simulink model "LKAS_AutoSave_20220223_1234"  (R2018b)
settings: Solver=FixedStepDiscrete  StartTime=0.0  StopTime=10.0  FixedStep=0.01  RelTol=1e-3
InitFcn:
  | tmpVer = ver('MATLAB');
  | tmpVer = str2num(tmpVer.Version);
  | % -------------------------------------------------------------------
  | %  MATLAB file generated by Simulink.saveVars on 21-Nov-2019 10:06:14
  | %  MATLAB version: 7.13.0.564 (R2011b)
  | % -------------------------------------------------------------------
  | 
  | 
  | SInt16 = Simulink.AliasType;
  | SInt16.Description = 'Num';
  | if (tmpVer > 7.11)
  | 	SInt16.DataScope = 'Auto';
  | end
  | SInt16.HeaderFile = 'Rte_Type.h';
  | SInt16.BaseType = 'int16';
  | 
  | SInt32 = Simulink.AliasType;
  | SInt32.Description = 'Num';
  | if (tmpVer > 7.11)
  | 	SInt32.DataScope = 'Auto';
  | end
  | SInt32.HeaderFile = 'Rte_Type.h';
  | SInt32.BaseType = 'int32';
  | 
  | SInt8 = Simulink.AliasType;
  | SInt8.Description = 'Num';
  | if (tmpVer > 7.11)
  | 	SInt8.DataScope = 'Auto';
  | end
  | SInt8.HeaderFile = 'Rte_Type.h';
  | SInt8.BaseType = 'int8';
  | 
  | T_A_m2_1024_1_u32 = Simulink.NumericType;
  | T_A_m2_1024_1_u32.Description = 'm2 (square meters  (m2))';
  | if (tmpVer > 7.11)
  | 	T_A_m2_1024_1_u32.DataScope = 'Auto';
  | end
  | T_A_m2_1024_1_u32.HeaderFile = 'Rte_Type.h';
  | T_A_m2_1024_1_u32.DataTypeMode = 'Fixed-point: slope and bias scaling';
  | T_A_m2_1024_1_u32.SignednessBool = false;
  | T_A_m2_1024_1_u32.WordLength = 32;
  | T_A_m2_1024_1_u32.FixedExponent = -10;
  | T_A_m2_1024_1_u32.SlopeAdjustmentFactor = 1;
  | T_A_m2_1024_1_u32.Bias = 0;
  | T_A_m2_1024_1_u32.DataTypeOverride = 'Inherit';
  | T_A_m2_1024_1_u32.IsAlias = true;
  | 
  | T_A_m2_65536_1_u16 = Simulink.NumericType;
  | T_A_m2_65536_1_u16.Description = 'm2 (square meters  (m2))';
  | if (tmpVer > 7.11)
  | 	T_A_m2_65536_1_u16.DataScope = 'Auto';
  | end
  | T_A_m2_65536_1_u16.HeaderFile = 'Rte_Type.h';
  | T_A_m2_65536_1_u16.DataTypeMode = 'Fixed-point: slope and bias scaling';
  | T_A_m2_65536_1_u16.SignednessBool = false;
  | T_A_m2_65536_1_u16.WordLength = 16;
  | T_A_m2_65536_1_u16.FixedExponent = -16;
  | T_A_m2_65536_1_u16.SlopeAdjustmentFactor = 1;
  | T_A_m2_65536_1_u16.Bias = 0;
  | T_A_m2_65536_1_u16.DataTypeOverride = 'Inherit';
  | ... (+4647 lines)
StopFcn:
  | clear  T_A_m2_1024_1_u32 T_A_m2_65536_1_u16 T_A_m2_Float32 T_A_mm2_10_1_u16 T_A_mm2_4_1_s16 T_A_mm2_Float32 T_Cnt_Num_10_1_u32 T_Cnt_Num_1_1_s16 T_Cnt_Num_1_1_s32 T_Cnt_Num_1_1_s8 T_Cnt_Num_1_1_u16 T_Cnt_Num_1_1_u32 T_Cnt_Num_1_1_u8 T_E_J_1_1_s32 T_E_J_Float32 T_E_kJ_128_1_s32 T_E_kJ_Float32 T_E_kwh_10_1_u16 T_E_kwh_Float32 T_Epl_kwhpkm_100_1_u16 T_Epl_kwhpkm_Float32 T_F_N_1_1_s16 T_F_N_Float32 T_I_A_1000_1_u16 T_I_A_1048576_1_s32 T_I_A_2048_1_s16 T_I_A_32_1_s16 T_I_A_Float32 T_I_mA_1_1_s16 T_I_mA_32768_128_s16 T_I_mA_Float32 T_J_kgpm2_128_1_u16 T_J_kgpm2_Float32 T_K_NA_1000_1_s16 T_K_NA_100_1_s16 T_K_NA_100_1_u16 T_K_NA_1024_1_s16 T_K_NA_1024_1_u16 T_K_NA_128_1_s16 T_K_NA_128_1_u16 T_K_NA_128_1_u8 T_K_NA_16777216_1_u32 T_K_NA_16_1_s16 T_K_NA_16_1_u16 T_K_NA_16_1_u8 T_K_NA_1_16_u16 T_K_NA_1_1_s16 T_K_NA_1_1_u16 T_K_NA_1_1_u8 T_K_NA_32768_1_s16 T_K_NA_32768_1_u16 T_K_NA_32_1_s8 T_K_NA_4096_1_u16 T_K_NA_4194304_1_s32 T_K_NA_4194304_1_u16 T_K_NA_65536_1_s32 T_K_NA_65536_1_u16 T_K_NA_8192_1_s16 T_K_NA_8_1_s16 T_K_NA_Float32 T_M_Nm_16_1_s16 T_M_Nm_1_1_s16 T_M_Nm_32768_1_s16 T_M_Nm_32_1_s16 T_M_Nm_4_1_s16 T_M_Nm_512_1_s16 T_M_Nm_Float32 T_P_W_1_4_s16 T_P_W_1_8_s16 T_P_W_Float32 T_P_kW_128_1_s16 T_P_kW_1_8_s16 T_P_kW_8_1_s32 T_P_kW_Float32 T_Pct_pct_1024_1_s32 T_Pct_pct_1024_1_u32 T_Pct_pct_10_1_s16 T_Pct_pct_10_1_u32 T_Pct_pct_128_100_s8 T_Pct_pct_1_1_s16 T_Pct_pct_1_4_u8 T_Pct_pct_255_100_u16 T_Pct_pct_255_100_u8 T_Pct_pct_256_1_s16 T_Pct_pct_256_1_u16 T_Pct_pct_65535_100_u16 T_Pct_pct_Float32 T_R_ohm_1024_1_s16 T_R_ohm_32_1_s16 T_R_ohm_Float32 T_TK_K_16_1_s16 T_TK_K_Float32 T_T_degC_10_400_1_u16 T_T_degC_16_1_s16 T_T_degC_1_40_1_u8 T_T_degC_2_80_1_u8 T_T_degC_Float32 T_U_V_1000_1_u16 T_U_V_10_1_u8 T_U_V_200_1_u8 T_U_V_32_1_s16 T_U_V_4096_1_s16 T_U_V_512_1_s16 T_U_V_65535_8_u16 T_U_V_8192_1_u16 T_U_V_Float32 T_U_mV_1_1_s16 T_U_mV_256_20_u16 T_U_mV_Float32 T_V_l_256_1_s16 T_V_l_4096_1_s16 T_V_l_64_1_s16 T_V_l_65535_100_u16 T_V_l_Float32 T_V_ml_128_1_s16 T_V_ml_1_1_s16 T_V_ml_32768_1_s16 T_V_ml_Float32 T_V_ul_32_1_u16 T_V_ul_Float32 T_Vpl_clpkm_512_1_u16 T_Vpl_clpkm_Float32 T_a_kphps_16_1_s16 T_a_kphps_Float32 T_a_mps2_128_1_s16 T_a_mps2_Float32 T_c_MJpkg_256_1_s16 T_c_MJpkg_Float32 T_c_kJpgpK_1024_1_s16 T_c_kJpgpK_Float32 T_c_kJpkgpK_128_1_u16 T_c_kJpkgpK_Float32 T_chrg_Ah_1_1_s16 T_chrg_Ah_1_1_u16 T_chrg_Ah_1_1_u8 T_chrg_Ah_256_1_u16 T_chrg_Ah_4194304_1_s32 T_chrg_Ah_512_1_u16 T_chrg_Ah_8_1_u16 T_chrg_Ah_Float32 T_cmp_NA_100_1_s16 T_cmp_NA_128_1_s16 T_cmp_NA_16_1_s16 T_cmp_NA_32768_1_u16 T_cmp_NA_Float32 T_d2n_rpmps2_4_1_s16 T_d2n_rpmps2_Float32 T_dPct_pctps_16_1_s16 T_dPct_pctps_256_1_s16 T_dPct_pctps_Float32 T_dT_degCps_128_1_s16 T_dT_degCps_Float32 T_dV_lph_1_1_s16 T_dV_lph_Float32 T_dV_lpm_128_1_s16 T_dV_lpm_32_1_s16 T_dV_lpm_Float32 T_dV_lps_1024_1_u16 T_dV_lps_4_1_u16 T_dV_lps_Float32 T_dV_mlps_1024_1_s16 T_dV_mlps_Float32 T_d_BitField16 T_dm_gps_128_1_s16 T_dm_gps_128_1_u16 T_dm_gps_256_1_u16 T_dm_gps_Float32 T_dm_mgps_1_1_s16 T_dm_mgps_Float32 T_dn_rpmps_1_1_s16 T_dn_rpmps_2_1_s16 T_dn_rpmps_Float32 T_dp_Paps_1_1_s16 T_dp_Paps_Float32 T_dp_kPaps_1_1_s16 T_dp_kPaps_8_1_s16 T_dp_kPaps_Float32 T_dphi_degps_128_1_s16 T_dphi_degps_8_1_s16 T_dphi_degps_Float32 T_dr_ps_256_1_s16 T_dr_ps_Float32 T_drho_mgplps_1_2_s16 T_drho_mgplps_Float32 T_e_NA_1_1_u8 T_f_Hz_1_1_u16 T_f_Hz_1_1_u32 T_f_Hz_64_1_u16 T_f_Hz_8_1_s16 T_f_Hz_Float32 T_g_BitField32 T_l_km_16_1_s16 T_l_km_1_1_u16 T_l_km_1_1_u32 T_l_km_Float32 T_l_m_1024_1_s16 T_l_m_16_1_s16 T_l_m_1_1_u32 T_l_m_Float32 T_l_mm_16_1_s16 T_l_mm_1_1_u16 T_l_mm_4096_1_s16 T_l_mm_4_1_u8 T_l_mm_64_1_s16 T_l_mm_Float32 T_m_g_1_1_s16 T_m_g_2048_1_s16 T_m_g_32_1_u16 T_m_g_Float32 T_m_kg_1024_1_s16 T_m_kg_1_1_s16 T_m_kg_1_1_u32 T_m_kg_Float32 T_m_mg_128_1_s16 T_m_mg_32_1_s16 T_m_mg_Float32 T_n_rpm_1_1_s16 T_n_rpm_1_25_u8 T_n_rpm_256_50_u16 T_n_rpm_2_25_u8 T_n_rpm_4_1_u16 T_n_rpm_Float32 T_p_MPa_64_1_s16 T_p_MPa_Float32 T_p_Pa_1_1_s16 T_p_Pa_Float32 T_p_kPa_1_10_u16 T_p_kPa_1_1_s16 T_p_kPa_1_1_u8 T_p_kPa_256_1_u16 T_p_kPa_32_1_u16 T_p_kPa_64_1_s16 T_p_kPa_Float32 T_phi_deg_100_1_s16 T_phi_deg_1024_1_s16 T_phi_deg_128_1_s16 T_phi_deg_1_1_u8 T_phi_deg_256_1_s16 T_phi_deg_2_1_s8 T_phi_deg_32_1_s16 T_phi_deg_512_6_s32 T_phi_deg_Float32 T_phi_rad_2048_1_s16 T_phi_rad_Float32 T_r_NA_1024_1_s16 T_r_NA_1024_1_u16 T_r_NA_16384_1_s16 T_r_NA_16_1_s16 T_r_NA_256_1_s8 T_r_NA_256_1_u16 T_r_NA_32768_1_u16 T_r_NA_32_1_u16 T_r_NA_4096_1_s16 T_r_NA_65535_2_u16 T_r_NA_8192_1_u16 T_r_NA_Float32 T_rho_gpl_8192_1_s16 T_rho_gpl_Float32 T_rho_kgpm3_16_1_s16 T_rho_kgpm3_Float32 T_rho_mgpl_1_1_s16 T_rho_mgpl_64_1_s16 T_rho_mgpl_Float32 T_t_hour_1_1_s16 T_t_hour_Float32 T_t_m_1_1_u16 T_t_m_Float32 T_t_ms_1_1_s16 T_t_ms_1_1_u16 T_t_ms_1_1_u32 T_t_ms_4096_1_s16 T_t_ms_64_1_s16 T_t_ms_Float32 T_t_s_1000_1_s16 T_t_s_100_1_s16 T_t_s_10_1_s16 T_t_s_10_1_u16 T_t_s_1_1_s16 T_t_s_1_1_u16 T_t_s_1_1_u32 T_t_s_Float32 T_t_us_10_1_u32 T_t_us_1_1_s16 T_t_us_1_1_u32 T_t_us_1_4_u16 T_t_us_Float32 T_v_kph_1_1_u8 T_v_kph_64_1_s16 T_v_kph_64_1_u16 T_v_kph_Float32 T_v_mps_256_1_s16 T_v_mps_Float32 T_w_radps_32_1_s16 T_w_radps_Float32 T_y_BitField8 T_y_BitFieldDiagProgress T_y_BitFieldDiagStatus T_y_NA_1_1_u8 SInt16 SInt32 SInt8 T_BOOLEAN UInt16 UInt32 UInt8 s16 s32 s8 u16 u32 u8
model workspace (MAT data in the model file):
  MCOS : class17 (value not decoded)
  MCOS : class17 (value not decoded)
  MCOS : class17 (value not decoded)
  MCOS : class17 (value not decoded)
  MCOS : class17 (value not decoded)
  MCOS : class17 (value not decoded)
  MCOS : class17 (value not decoded)
  MCOS : class17 (value not decoded)
  MCOS : class17 (value not decoded)
  MCOS : class17 (value not decoded)
  MCOS : class17 (value not decoded)
  MCOS : class17 (value not decoded)
  MCOS : class17 (value not decoded)
  MCOS : class17 (value not decoded)
  MCOS : class17 (value not decoded)
  MCOS : class17 (value not decoded)
  MCOS : class17 (value not decoded)
  MCOS : class17 (value not decoded)
  MCOS : class17 (value not decoded)
  MCOS : class17 (value not decoded)
  MCOS : class17 (value not decoded)
  MCOS : class17 (value not decoded)
  MCOS : class17 (value not decoded)
  MCOS : class17 (value not decoded)
  MCOS : class17 (value not decoded)
  MCOS : class17 (value not decoded)
  MCOS : class17 (value not decoded)
  MCOS : class17 (value not decoded)
  MCOS : class17 (value not decoded)
  MCOS : class17 (value not decoded)
  MCOS : class17 (value not decoded)
  MCOS : class17 (value not decoded)
  MCOS : class17 (value not decoded)
  MCOS : class17 (value not decoded)
  MCOS : class17 (value not decoded)
  MCOS : class17 (value not decoded)
  MCOS : class17 (value not decoded)
  MCOS : class17 (value not decoded)
  MCOS : class17 (value not decoded)
  MCOS : class17 (value not decoded)
  MCOS : class17 (value not decoded)
  MCOS : class17 (value not decoded)
  MCOS : class17 (value not decoded)
  MCOS : class17 (value not decoded)
  MCOS : class17 (value not decoded)
  MCOS : class17 (value not decoded)
  MCOS : class17 (value not decoded)
  MCOS : class17 (value not decoded)
  MCOS : class17 (value not decoded)
  MCOS : class17 (value not decoded)
  MCOS : class17 (value not decoded)
  MCOS : class17 (value not decoded)
  MCOS : class17 (value not decoded)
  MCOS : class17 (value not decoded)
  MCOS : class17 (value not decoded)
  MCOS : class17 (value not decoded)
  MCOS : class17 (value not decoded)
  MCOS : class17 (value not decoded)
  MCOS : class17 (value not decoded)
  MCOS : class17 (value not decoded)
  MCOS : class17 (value not decoded)
  MCOS : class17 (value not decoded)
  MCOS : class17 (value not decoded)
  MCOS : class17 (value not decoded)
  MCOS : class17 (value not decoded)
  MCOS : class17 (value not decoded)
  MCOS : class17 (value not decoded)
  MCOS : class17 (value not decoded)
  MCOS : class17 (value not decoded)
  MCOS : class17 (value not decoded)
  MCOS : class17 (value not decoded)
  MCOS : class17 (value not decoded)
  MCOS : class17 (value not decoded)
  MCOS : class17 (value not decoded)
  MCOS : class17 (value not decoded)
  MCOS : class17 (value not decoded)
  MCOS : class17 (value not decoded)
  MCOS : class17 (value not decoded)
  MCOS : class17 (value not decoded)
  MCOS : class17 (value not decoded)
  MCOS : class17 (value not decoded)
  MCOS : class17 (value not decoded)
  MCOS : class17 (value not decoded)
  MCOS : class17 (value not decoded)
  MCOS : class17 (value not decoded)
  MCOS : class17 (value not decoded)
  MCOS : class17 (value not decoded)
  MCOS : class17 (value not decoded)
  MCOS : class17 (value not decoded)
  MCOS : class17 (value not decoded)
  MCOS : class17 (value not decoded)
  MCOS : class17 (value not decoded)
  MCOS : class17 (value not decoded)
  MCOS : class17 (value not decoded)
  MCOS : class17 (value not decoded)
  MCOS : class17 (value not decoded)
  MCOS : class17 (value not decoded)
  MCOS : class17 (value not decoded)
  MCOS : class17 (value not decoded)
  MCOS : class17 (value not decoded)
  MCOS : class17 (value not decoded)
  MCOS : class17 (value not decoded)
undefined symbols (not defined in the file): LKA_CarWidth, LKA_SampleTime, LKA_StrRatio_C, LKA_Veh2CamL_C, LKA_Veh2CamW_C, LKA_WhlBaseL_C, LL_CompHdAg_C, LL_CompSWA_C, LL_CrvtPrvwT_C, LL_DesDvt_C, LL_DvtComp_C, LL_DvtPrvwT_C, LL_DvtSpdDet_vDvtSpdMin_C, LL_HandsOff_ExitTime, LL_HandsOff_TextTime, LL_HandsOff_WarnTime, LL_HdAgExT_C, LL_HdAgPrvwT_C, LL_LAccMax_C, LL_LAccRMax_C, LL_LDW_EarliestWarnLine_C, LL_LDW_LatestWarnLine_C, LL_LDWS_SUPPRESS_HEADING, LL_LFClb_TFC_FfCtlRatio_C, LL_LFClb_TFC_KdBalance_C, LL_LFClb_TFC_KdMaxSWA_C, LL_LFClb_TFC_KdV1_C, LL_LFClb_TFC_KdV2_C, LL_LFClb_TFC_KdVehSpdLwr_C, LL_LFClb_TFC_KdVehSpdUpr_C, LL_LFClb_TFC_Ki_C, LL_LFClb_TFC_KiMaxSWA_C, LL_LFClb_TFC_Kp_C, LL_LFClb_TFC_KpKlat_C, LL_LFClb_TFC_KpV1_C, LL_LFClb_TFC_KpV2_C, LL_LFClb_TFC_KpVehSpdLwr_C, LL_LFClb_TFC_KpVehSpdUpr_C, LL_LFClb_TFC_PrvwT_C, LL_LKA_EarliestWarnLine_C, LL_LKA_LatestWarnLine_C, LL_LKAExPrcs_ExitC0Dvt, LL_LKAExPrcs_ExitC0Swt, LL_LKAExPrcs_tiExitTime1, LL_LKAExPrcs_tiExitTime2, LL_LKAExPrcs_tiExitTime3, LL_LKAS_OUT_OF_CONTROL_LAT_VEL, LL_LKAS_OUT_OF_CONTROL_TTLC, LL_LKASWASyn_M0, LL_LKASWASyn_M1, LL_LKASWASyn_M2, LL_LKASWASyn_M3K, LL_LKASWASyn_SWAaddMax, LL_LKASWASyn_T2, LL_LKASWASyn_tiTrqSwaRtTime, LL_LKASWASyn_tiTrqSwaTime, LL_LKASWASyn_TrqMax, LL_LKASWASyn_TrqSwaAddSwt, LL_LKASWASyn_TrqSwaRateDiff, LL_LSpdCompT_C ... (+43)
libraries: simulink x138, canmsglib x8, dspstat3 x3, simulink_extras x1
(part 8 of 20)

== system LKAS_AutoSave_20220223_1234/LKAS/LL/LLOn/LKA/Lane Following (LF) ==
  LF_bsInInfoSyn : Inport
  LF_bsLKAInPInfo : Inport  Port=2
  LF_bsLFClb : Inport  Port=3
  Preview Information Calculation (PIC) : Subsystem  Description=|
      | Block Name:Preview Information Calculation
      | Ab.: PIC
      | No.: 02.01
      | Rev: 00.00.01
      | Update Date: 19-3-28
  Trajectory Following Control (TFC) : Subsystem  Description=|
      | Block Name:Trajectory Following Control
      | Ab.: TFC
      | No.: 02.02
      | Rev: 00.00.01
      | Update Date: 19-3-28
  LF_phiFfLFSWACmd : Outport
  LF_phiPropSWACmd : Outport  Port=2
  LF_phiIntegSWACmd : Outport  Port=3
  LF_phiDiffSWACmd : Outport  Port=4
  wires:
  Trajectory Following Control (TFC)/4(TFC_phiDiffSWACmd) -> LF_phiDiffSWACmd/1
  Trajectory Following Control (TFC)/3(TFC_phiIntegSWACmd) -> LF_phiIntegSWACmd/1
  Trajectory Following Control (TFC)/2(TFC_phiPropSWACmd) -> LF_phiPropSWACmd/1
  LF_bsLFClb/1 -> Trajectory Following Control (TFC)/3(TFC_bsTFCClb)
  Preview Information Calculation (PIC)/1(PIC_bsPrvwInfo) -> Trajectory Following Control (TFC)/1(TFC_bsPrvwInfo)
  LF_bsInInfoSyn/1 -> Trajectory Following Control (TFC)/2(TFC_bsInInfoSyn)
  Trajectory Following Control (TFC)/1(TFC_phiFfSWACmd) -> LF_phiFfLFSWACmd/1
  LF_bsLKAInPInfo/1 -> Preview Information Calculation (PIC)/1(PIC_bsLKAInPInfo)

== system LKAS_AutoSave_20220223_1234/LKAS/LL/LLOn/LKA/Plan To LaneFollowing (PTLF) ==
  InP : Inport
  Plan : Inport  Port=2
  T1 : Inport  Port=3
  DrvTrq : Inport  Port=4
  Ff : Inport  Port=5
  P : Inport  Port=6
  I : Inport  Port=7
  D : Inport  Port=8
  Add1 : Sum  Inputs=+-
  Add2 : Sum  Inputs=+-
  Add3 : Sum
  Add4 : Sum  Inputs=+++++
  Add5 : Sum  Inputs=+-
  Bus Selector1 : BusSelector  OutputSignals=bsPrCrvtInfo.crPrvwCrvt
  Bus Selector2 : BusSelector  OutputSignals=bsHdAgInfo.L0_C1,bsHdAgInfo.R0_C1
  Constant1 : Constant  Value=0.1  OutDataTypeStr=single
  Constant2 : Constant  OutDataTypeStr=single
  Divide : Product  Inputs=*/
  Divide{1..2,5..7} (5 alike) : Product  Inputs=**
  Divide3 : Product  Inputs=*/
  Divide4 : Product  Inputs=*/
  InsideJudge : Subsystem
  InsideJudge1 : Subsystem
  LowPass : Subsystem
  Saturation : Saturate  UpperLimit=1  LowerLimit=0
      settings: AttributesFormatString="Min = %<LowerLimit>  Max = %<UpperLimit>"
  Saturation1 : Saturate  UpperLimit=1  LowerLimit=0
      settings: AttributesFormatString="Min = %<LowerLimit>  Max = %<UpperLimit>"
  Saturation2 : Saturate  UpperLimit=1  LowerLimit=0
      settings: AttributesFormatString="Min = %<LowerLimit>  Max = %<UpperLimit>"
  Saturation3 : Saturate  UpperLimit=0.004  LowerLimit=-0.004
      settings: AttributesFormatString="Min = %<LowerLimit>  Max = %<UpperLimit>"
  Saturation6 : Saturate  LowerLimit=0.2
      settings: AttributesFormatString="Min = %<LowerLimit>  Max = %<UpperLimit>"
  Switch : Switch  Criteria=u2 > Threshold
  TickTime (TTime) : Subsystem
      mask Display:
      | port_label('output', 1, 'TTime');
      | color('blue');
      | text(0.98,0.9,'VCDC Block','horizontalAlignment','right');
      | color('black');
      | text(0.5,0.55,'Tick Time','horizontalAlignment','center');
      | text(0.5,0.4,'(TTime)','horizontalAlignment','center');
  TimeGain : Subsystem
  SWACmd : Outport
  tag scope: LKA_SampleTime_Mon=global, T1_Mon=global
  wires:
  Constant1/1 -> LowPass/1(T)
  [LKA_SampleTime] -> [LKA_SampleTime_Mon], LowPass/3(dT)
  LowPass/1(y) -> SWACmd/1  "SWACmd"
  Divide2/1 -> Add4/3  "S_D"
  Divide4/1 -> Saturation1/1
  Divide1/1 -> Add4/2  "S_PI"
  Add3/1 -> Divide1/2
  I/1 -> Add3/2
  P/1 -> Add3/1
  Divide7/1 -> Add4/1  "S_Plan"
  DrvTrq/1 -> Divide6/1
  D/1 -> Divide2/1
  Ff/1 -> Divide5/2
  Add5/1 -> Divide7/2
  Divide6/1 -> Add4/5  "S_DT"
  [Plan] -> Divide7/1
  Saturation2/1 -> Divide1/1, Add5/2
  Constant2/1 -> Add5/1
  Saturation/1 -> Divide6/2
  Divide/1 -> Saturation2/1
  Divide3/1 -> Saturation/1
  [T1] -> Add2/2
  Add2/1 -> Divide/1
  Add4/1 -> LowPass/2(u)
  [TFC] -> Divide/2
  Saturation1/1 -> Divide2/2
  Bus Selector1/1 -> Saturation3/1  "<crPrvwCrvt>"
  Saturation3/1 -> InsideJudge/2(Crvt)
  Divide5/1 -> Switch/3, Switch/1
  TimeGain/1(Out1) -> Divide5/1
  TickTime (TTime)/1(Out1) -> [Time]
  [ActFlg] -> InsideJudge/1(Flg)
  InsideJudge/1(Out1) -> Switch/2
  Switch/1 -> Add4/4  "S_Ff"
  [Time] -> Divide3/1
  [Time] -> Add2/1
  [T1] -> Divide3/2
  InsideJudge1/1(T1_1) -> [T1_Mon], [T1], Saturation6/1
  Saturation6/1 -> [TFC]
  [Time] -> TimeGain/1(Time)
  [T1] -> TimeGain/2(T1)
  [TFC] -> TimeGain/3(TFC)
  [T1] -> Add1/2
  [TFC] -> Divide4/2
  Add1/1 -> Divide4/1
  [Time] -> Add1/1
  InP/1 -> Bus Selector2/1, Bus Selector1/1
  [ActFlg] -> InsideJudge1/1(Flg)
  Bus Selector2/1 -> InsideJudge1/2(HdAgLft)  "<L0_C1>"
  Bus Selector2/2 -> InsideJudge1/3(HdAgRgt)  "<R0_C1>"
  T1/1 -> InsideJudge1/4(T1)
  Plan/1 -> InsideJudge1/5(Plan)
  [Time] -> InsideJudge1/6(Time)
  InsideJudge1/2(Plan_1) -> [Plan]

== system LKAS_AutoSave_20220223_1234/LKAS/LL/LLOn/LKA Input Processing (LKAInP)/Curvature Calculation (Crvt) ==
  PrvwCrvt_bsInInfoSyn : Inport
  Add : Sum  AccumDataTypeStr=single
  Bus Creator1 : BusCreator  Inputs=3
  Bus Selector1 : BusSelector  OutputSignals=bsLaneInfo.bsL0Info.L0_C2,bsLaneInfo.bsR0Info.R0_C2
  Gain : Gain  Gain=0.5
  Crvt_bsCrvtInfo : Outport
  wires:
  Add/1 -> Gain/1
  Bus Selector1/1 -> Bus Creator1/2, Add/1  "<L0_C2>"
  Bus Selector1/2 -> Bus Creator1/3, Add/2  "<R0_C2>"
  PrvwCrvt_bsInInfoSyn/1 -> Bus Selector1/1
  Gain/1 -> Bus Creator1/1  "crCrvt"
  Bus Creator1/1 -> Crvt_bsCrvtInfo/1

== system LKAS_AutoSave_20220223_1234/LKAS/LL/LLOn/LKA Input Processing (LKAInP)/Deviation Calculation (Dvt) ==
  Dvt_bsInInfoSyn : Inport
  Dvt_bsLLClb : Inport  Port=2
  Add : Sum  AccumDataTypeStr=single
  Bus Creator1 : BusCreator  Inputs=3
  Bus Selector2 : BusSelector  OutputSignals=bsLaneInfo.bsL0Info.L0_C1,bsLaneInfo.bsL0Info.L0_C0,bsLaneInfo.bsR0Info.R0_C0,bsLaneInfo.bsR0Info.R0_C1
  Gain : Gain  Gain=0.5
  Left Front Conner Deviation Calculation (LFCDvtCalc) : Subsystem
  Right Front Conner Deviation Calculation (RFCDvtCalc) : Subsystem
  Dvt_bsDvtInfo : Outport
  wires:
  Bus Selector2/1 -> Left Front Conner Deviation Calculation (LFCDvtCalc)/1(LFCDvtCalc_bsHdAgInfo)  "<L0_C1>"
  Dvt_bsInInfoSyn/1 -> Bus Selector2/1
  Bus Creator1/1 -> Dvt_bsDvtInfo/1
  Bus Selector2/2 -> Left Front Conner Deviation Calculation (LFCDvtCalc)/2(LFCDvtCalc_lDvt)  "<L0_C0>"
  Bus Selector2/3 -> Right Front Conner Deviation Calculation (RFCDvtCalc)/1(RFCDvtCalc_lDvt)  "<R0_C0>"
  Left Front Conner Deviation Calculation (LFCDvtCalc)/1(DvtCalc_lLftDvt) -> Bus Creator1/1, Add/1  "ILftDvt"
  Right Front Conner Deviation Calculation (RFCDvtCalc)/1(DvtCalc_lRgtDvt) -> Add/2, Bus Creator1/3  "IRgtDvt"
  Bus Selector2/4 -> Right Front Conner Deviation Calculation (RFCDvtCalc)/2(RFCDvtCalc_bsHdAgInfo)  "<R0_C1>"
  Add/1 -> Gain/1
  Gain/1 -> Bus Creator1/2  "lDvt"
  Dvt_bsLLClb/1 -> Left Front Conner Deviation Calculation (LFCDvtCalc)/3(LFCDvtCalc_bsLLClb), Right Front Conner Deviation Calculation (RFCDvtCalc)/3(RFCDvtCalc_bsLLClb)

== system LKAS_AutoSave_20220223_1234/LKAS/LL/LLOn/LKA Input Processing (LKAInP)/Heading Angle Calculation (HdAg) ==
  HdAg_bsInInfoSyn : Inport
  Add : Sum  AccumDataTypeStr=single
  Bus Creator : BusCreator  Inputs=3
  Bus Selector : BusSelector  OutputSignals=bsLaneInfo.bsL0Info.L0_C1,bsLaneInfo.bsR0Info.R0_C1
  Gain : Gain  Gain=0.5
  HdAg_bsHdAgInfo : Outport
  wires:
  Bus Creator/1 -> HdAg_bsHdAgInfo/1
  Gain/1 -> Bus Creator/1  "phiHdAg"
  Bus Selector/2 -> Bus Creator/3, Add/2  "<R0_C1>"
  Bus Selector/1 -> Bus Creator/2, Add/1  "<L0_C1>"
  HdAg_bsInInfoSyn/1 -> Bus Selector/1
  Add/1 -> Gain/1

== system LKAS_AutoSave_20220223_1234/LKAS/LL/LLOn/LKA Input Processing (LKAInP)/Lane Width Calculation (LW) ==
  LW_bsInInfoSyn : Inport
  Abs : Abs
  Abs1 : Abs
  Add : Sum
  Bus Selector : BusSelector  OutputSignals=bsLaneInfo.bsL0Info.L0_C0,bsLaneInfo.bsR0Info.R0_C0
  Saturation : Saturate  UpperLimit=6  LowerLimit=2
      settings: AttributesFormatString="Min = %<LowerLimit>  Max = %<UpperLimit>"
  LW_LaneWidth : Outport
  wires:
  LW_bsInInfoSyn/1 -> Bus Selector/1
  Bus Selector/1 -> Abs/1  "<L0_C0>"
  Bus Selector/2 -> Abs1/1  "<R0_C0>"
  Abs/1 -> Add/1
  Abs1/1 -> Add/2
  Add/1 -> Saturation/1
  Saturation/1 -> LW_LaneWidth/1  "LaneWidth"

== system LKAS_AutoSave_20220223_1234/LKAS/LL/LLOn/LKA Input Processing (LKAInP)/Previewed Curvature Calculation (PrCrvt) ==
  PrvwCrvt_bsInInfoSyn : Inport
  PrvwCrvt_tiCrvtPrvwT_C : Inport  Port=2
  PrvwCrvt_stLKAActvFlg : Inport  Port=3
  Add1 : Sum  AccumDataTypeStr=single
  Bus Creator : BusCreator  Inputs=4
  Bus Selector : BusSelector  OutputSignals=bsLKAClb.LL_CrvtPrvwT_C
  Bus Selector2 : BusSelector  OutputSignals=bsLaneInfo.bsL0Info,bsVehMovInfo.ESC_VehSpd,bsLaneInfo.bsR0Info
  Curvature Ahead of Left Lane Line (CrvtAhdLft) : Subsystem
  Curvature Ahead of Left Lane Line (CrvtAhdLft)1 : Subsystem
  Gain1 : Gain  Gain=0.5
  Lane Information Selection (LaneInfoSel) : Subsystem
  Z Calculation (ZCalc) : Subsystem
  PrvwCrvt_bsPrvwCrvtInfo : Outport
  wires:
  PrvwCrvt_bsInInfoSyn/1 -> Bus Selector2/1
  Z Calculation (ZCalc)/1(ZCalc_lPrvwDstZ) -> Curvature Ahead of Left Lane Line (CrvtAhdLft)1/1(CrvtAhdRgt_lPrvwDstZ), Curvature Ahead of Left Lane Line (CrvtAhdLft)/2(CrvtAhdLft_lPrvwDstZ)
  Bus Selector2/1 -> Curvature Ahead of Left Lane Line (CrvtAhdLft)/1(CrvtAhdLft_bsL0Info)  "<bsL0Info>"
  Bus Selector2/3 -> Curvature Ahead of Left Lane Line (CrvtAhdLft)1/2(CrvtAhdRgt_bsR0Info)  "<bsR0Info>"
  Bus Selector2/2 -> Z Calculation (ZCalc)/1(ZCalc_vVehSpd)  "<ESC_VehSpd>"
  PrvwCrvt_tiCrvtPrvwT_C/1 -> Bus Selector/1
  Bus Selector/1 -> Z Calculation (ZCalc)/2(ZCalc_tiCrvtPrvwT_C)  "<LL_CrvtPrvwT_C>"
  Bus Creator/1 -> PrvwCrvt_bsPrvwCrvtInfo/1
  Gain1/1 -> Bus Creator/4  "crPrvwCrvtMean"
  Add1/1 -> Gain1/1
  Lane Information Selection (LaneInfoSel)/1(LaneInfoSel_facmActvLane) -> Bus Creator/1  "crPrvwCrvt"
  Curvature Ahead of Left Lane Line (CrvtAhdLft)1/1(CrvtAhdRgt_crCrvtAhdRgt) -> Add1/2, Lane Information Selection (LaneInfoSel)/3(LaneInfoSel_facmRgtLane), Bus Creator/3  "crPrvwCrvtRgt"
  Curvature Ahead of Left Lane Line (CrvtAhdLft)/1(CrvtAhdLft_crCrvtAhdLft) -> Lane Information Selection (LaneInfoSel)/2(LaneInfoSel_facmLftLane), Bus Creator/2, Add1/1  "crPrvwCrvtLft"
  PrvwCrvt_stLKAActvFlg/1 -> Lane Information Selection (LaneInfoSel)/1(LaneInfoSel_stLKAActvFlg)

== system LKAS_AutoSave_20220223_1234/LKAS/LL/LLOn/LKA Input Processing (LKAInP)/Previewed Deviation Calculation (PrDvt) ==
  PrdcDvt_bsLLClb : Inport
  PrvwDvt_bsInInfoSyn : Inport  Port=2
  Add1 : Sum  AccumDataTypeStr=single
  Bus Creator1 : BusCreator  Inputs=3
  Bus Selector : BusSelector  OutputSignals=bsLaneInfo.bsL0Info,bsVehMovInfo.ESC_VehSpd,bsLaneInfo.bsR0Info
  Bus Selector1 : BusSelector  OutputSignals=bsLKAClb.LL_DvtPrvwT_C
  Gain1 : Gain  Gain=0.5
  Previewed Deviation of Left Lane Line (PrvwDvtLft) : Subsystem
  Previewed Deviation of Right Lane Line (PrvwDvtRgt) : Subsystem
  Z Calculation (ZCalc) : Subsystem
  PrvwDvt_bsPrvwDvtInfo : Outport
  wires:
  Bus Selector1/1 -> Z Calculation (ZCalc)/2(ZCalc_tiDvtPrvwT_C)  "<LL_DvtPrvwT_C>"
  PrdcDvt_bsLLClb/1 -> Bus Selector1/1
  Bus Selector/1 -> Previewed Deviation of Left Lane Line (PrvwDvtLft)/1(PrdcDvtLft_bsL0Info)  "<bsL0Info>"
  PrvwDvt_bsInInfoSyn/1 -> Bus Selector/1
  Z Calculation (ZCalc)/1(ZCalc_lPrvwDstZ) -> Previewed Deviation of Right Lane Line (PrvwDvtRgt)/1(PrdcDvtRgt_lPrvwDstZ), Previewed Deviation of Left Lane Line (PrvwDvtLft)/2(PrdcDvtLft_lPrvwDstZ)
  Previewed Deviation of Right Lane Line (PrvwDvtRgt)/1(PrvwDvtRgt_lPrvwDvtRgt) -> Bus Creator1/2, Add1/2  "lPrvwDvtRgt"
  Bus Selector/2 -> Z Calculation (ZCalc)/1(ZCalc_vVehSpd)  "<ESC_VehSpd>"
  Bus Selector/3 -> Previewed Deviation of Right Lane Line (PrvwDvtRgt)/2(PrdcDvtRgt_bsR0Info)  "<bsR0Info>"
  Previewed Deviation of Left Lane Line (PrvwDvtLft)/1(PrvwDvtLft_lPrvwDvtLft) -> Bus Creator1/1, Add1/1  "lPrvwDvtLft"
  Bus Creator1/1 -> PrvwDvt_bsPrvwDvtInfo/1
  Gain1/1 -> Bus Creator1/3  "lPrvwDvtMean"
  Add1/1 -> Gain1/1

== system LKAS_AutoSave_20220223_1234/LKAS/LL/LLOn/LKA Input Processing (LKAInP)/Previewed Heading Angle Calculation (PrHdAg) ==
  PrHdAg_bsInInfoSyn : Inport
  PrHdAg_bsLLClb : Inport  Port=2
  PrHdAg_bsTTLCInfo : Inport  Port=3
  Add1 : Sum  AccumDataTypeStr=single
  Add2 : Sum  AccumDataTypeStr=single
  Bus Creator1 : BusCreator  Inputs=4
  Bus Selector2 : BusSelector  OutputSignals=bsLaneInfo.bsL0Info,bsVehMovInfo.ESC_VehSpd,bsLaneInfo.bsR0Info
  Bus Selector3 : BusSelector  OutputSignals=bsLKAClb.LL_HdAgPrvwT_C
  Bus Selector4 : BusSelector  OutputSignals=LFTTTLC,RGTTTLC
  Compare To Constant : simulink/Logic and Bit Operations/Compare To Constant  relop=<=  const=2  OutDataTypeStr=boolean
  Compare To Constant1 : simulink/Logic and Bit Operations/Compare To Constant  relop=<=  const=2  OutDataTypeStr=boolean
  Gain1 : Gain  Gain=0.5
  Gain2 : Gain  Gain=0.5
  Perdicted Heading Angle from Right Lane Line (PrdcHdAgRgt) : Subsystem
  Perdicted Heading Angle from Right Lane Line (PrdcHdAgRgt)1 : Subsystem
  Predicted Heading Angle from Left Lane Line (PrdcHdAgtLft) : Subsystem
  Predicted Heading Angle from Left Lane Line (PrdcHdAgtLft)1 : Subsystem
  Saturation : Saturate  UpperLimit=2  LowerLimit=0.5
      settings: AttributesFormatString="Min = %<LowerLimit>  Max = %<UpperLimit>"
  Saturation1 : Saturate  UpperLimit=2  LowerLimit=0.5
      settings: AttributesFormatString="Min = %<LowerLimit>  Max = %<UpperLimit>"
  Switch : Switch  Criteria=u2 > Threshold
  Switch1 : Switch  Criteria=u2 > Threshold
  Z Calculation (ZCalc) : Subsystem
  Z Calculation (ZCalc)1 : Subsystem
  PrHdAg_bsPrHdAgInfo : Outport
  wires:
  PrHdAg_bsInInfoSyn/1 -> Bus Selector2/1
  Bus Selector2/3 -> Perdicted Heading Angle from Right Lane Line (PrdcHdAgRgt)1/2(PrdcHdAgRgt_bsR0Info), Perdicted Heading Angle from Right Lane Line (PrdcHdAgRgt)/2(PrdcHdAgRgt_bsR0Info)  "<bsR0Info>"
  Z Calculation (ZCalc)/1(ZCalc_lPrvwDstZ) -> Add1/1, Predicted Heading Angle from Left Lane Line (PrdcHdAgtLft)/2(PrdcHdAgtLft_lPrvwDstZ)
  Bus Selector4/1 -> Switch/1, Compare To Constant/1  "<LFTTTLC>"
  Bus Selector2/1 -> Predicted Heading Angle from Left Lane Line (PrdcHdAgtLft)1/1(PrdcHdAgtLft_bsL0Info), Predicted Heading Angle from Left Lane Line (PrdcHdAgtLft)/1(PrdcHdAgtLft_bsL0Info)  "<bsL0Info>"
  Saturation/1 -> Z Calculation (ZCalc)/2(ZCalc_tiHdAgPrvwT_C)
  PrHdAg_bsTTLCInfo/1 -> Bus Selector4/1
  Bus Creator1/1 -> PrHdAg_bsPrHdAgInfo/1
  Bus Selector4/2 -> Switch1/1, Compare To Constant1/1  "<RGTTTLC>"
  Predicted Heading Angle from Left Lane Line (PrdcHdAgtLft)/1(PrdcHdAgtLft_phiPrdcHdAgLft) -> Bus Creator1/1  "phiPrvwTTLCHdAgLft"
  Perdicted Heading Angle from Right Lane Line (PrdcHdAgRgt)/1(PrdcHdAgRgt_phiPrdcHdAgRgt) -> Bus Creator1/2  "phiPrvwTTLCHdAgRgt"
  Bus Selector2/2 -> Z Calculation (ZCalc)1/1(ZCalc_vVehSpd), Z Calculation (ZCalc)/1(ZCalc_vVehSpd)  "<ESC_VehSpd>"
  Add2/1 -> Gain2/1
  Gain2/1 -> Bus Creator1/3  "phiPrvwHdAgMean"
  PrHdAg_bsLLClb/1 -> Bus Selector3/1
  Compare To Constant/1 -> Switch/2
  Switch/1 -> Saturation/1
  Switch1/1 -> Saturation1/1
  Bus Selector3/1 -> Switch/3, Switch1/3  "<LL_HdAgPrvwT_C>"
  Saturation1/1 -> Z Calculation (ZCalc)1/2(ZCalc_tiHdAgPrvwT_C)
  Z Calculation (ZCalc)1/1(ZCalc_lPrvwDstZ) -> Add1/2, Perdicted Heading Angle from Right Lane Line (PrdcHdAgRgt)/1(PrdcHdAgRgt_lPrvwDstZ)
  Compare To Constant1/1 -> Switch1/2
  Add1/1 -> Gain1/1
  Gain1/1 -> Predicted Heading Angle from Left Lane Line (PrdcHdAgtLft)1/2(PrdcHdAgtLft_lPrvwDstZ), Perdicted Heading Angle from Right Lane Line (PrdcHdAgRgt)1/1(PrdcHdAgRgt_lPrvwDstZ), Bus Creator1/4  "PrvwZMean"
  Predicted Heading Angle from Left Lane Line (PrdcHdAgtLft)1/1(PrdcHdAgtLft_phiPrdcHdAgLft) -> Add2/1  "phiPrvwTTLCHdAgLft"
  Perdicted Heading Angle from Right Lane Line (PrdcHdAgRgt)1/1(PrdcHdAgRgt_phiPrdcHdAgRgt) -> Add2/2  "phiPrvwTTLCHdAgRgt"

== system LKAS_AutoSave_20220223_1234/LKAS/LL/LLOn/LKA Input Processing (LKAInP)/Steering Wheel Position Calculation (SWAPosCal) ==
  SWAPosCal_bsInInfoSyn : Inport
  SWAPosCal_bsLLClb : Inport  Port=2
  Bus Selector : BusSelector  OutputSignals=bsLaneInfo.bsL0Info,bsLaneInfo.bsR0Info,bsVehMovInfo.ESC_VehSpd,bsSWAInfo.SW_Angle
  Bus Selector2 : BusSelector  OutputSignals=bsConstantClb.LKA_SampleTime
  Subsystem : Subsystem
  Subsystem1 : Subsystem
  SWAPosCal : Outport
  wires:
  SWAPosCal_bsInInfoSyn/1 -> Bus Selector/1
  Bus Selector/1 -> Subsystem1/1(L0)  "<bsL0Info>"
  Bus Selector/2 -> Subsystem1/2(R0)  "<bsR0Info>"
  Subsystem1/1(Flg) -> Subsystem/Enable  "SWAPosEna"
  Bus Selector/3 -> Subsystem1/3(VehSpd)  "<ESC_VehSpd>"
  Bus Selector/4 -> Subsystem1/4(SWA), Subsystem/1(SWAIn)  "<SW_Angle>"
  Subsystem/1(SWAPos) -> SWAPosCal/1
  SWAPosCal_bsLLClb/1 -> Bus Selector2/1
  Bus Selector2/1 -> Subsystem1/5(LKA_SampleTime), Subsystem/2(LKA_SampleTime)  "<LKA_SampleTime>"

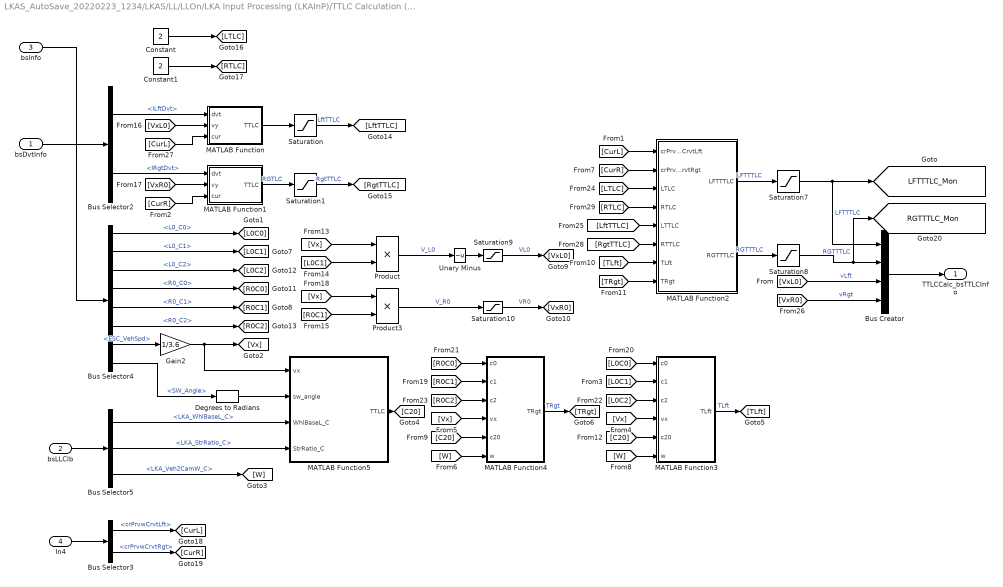
== system LKAS_AutoSave_20220223_1234/LKAS/LL/LLOn/LKA Input Processing (LKAInP)/TTLC Calculation (TTLCCalc) ==
  bsDvtInfo : Inport
  bsLLClb : Inport  Port=2
  bsInfo : Inport  Port=3
  In4 : Inport  Port=4
  Bus Creator : BusCreator  Inputs=4
  Bus Selector2 : BusSelector  OutputSignals=ILftDvt,IRgtDvt
  Bus Selector3 : BusSelector  OutputSignals=crPrvwCrvtLft,crPrvwCrvtRgt
  Bus Selector4 : BusSelector  OutputSignals=bsLaneInfo.bsL0Info.L0_C0,bsLaneInfo.bsL0Info.L0_C1,bsLaneInfo.bsL0Info.L0_C2,bsLaneInfo.bsR0Info.R0_C0,bsLaneInfo.bsR0Info.R0_C1,bsLaneInfo.bsR0Info.R0_C2,bsVehMovInfo.ESC_VehSpd,bsSWAInfo.SW_Angle
  Bus Selector5 : BusSelector  OutputSignals=bsConstantClb.LKA_WhlBaseL_C,bsConstantClb.LKA_StrRatio_C,bsConstantClb.LKA_Veh2CamW_C
  Constant : Constant  Value=2  OutDataTypeStr=single
  Constant1 : Constant  Value=2  OutDataTypeStr=single
  Degrees to Radians : simulink_extras/Transformations/Degrees to Radians
  Gain2 : Gain  Gain=1/3.6
  MATLAB Function : MATLAB Function  TreatAsAtomicUnit=on
  MATLAB Function1 : MATLAB Function  TreatAsAtomicUnit=on
  MATLAB Function2 : MATLAB Function  TreatAsAtomicUnit=on
  MATLAB Function3 : MATLAB Function  TreatAsAtomicUnit=on
  MATLAB Function4 : MATLAB Function  TreatAsAtomicUnit=on
  MATLAB Function5 : MATLAB Function  TreatAsAtomicUnit=on
  Product : Product
  Product3 : Product
  Saturation : Saturate  UpperLimit=2  LowerLimit=0.6  OutDataTypeStr=single
      settings: AttributesFormatString="Min = %<LowerLimit>  Max = %<UpperLimit>"
  Saturation1 : Saturate  UpperLimit=2  LowerLimit=0.6  OutDataTypeStr=single
      settings: AttributesFormatString="Min = %<LowerLimit>  Max = %<UpperLimit>"
  Saturation10 : Saturate  UpperLimit=2  LowerLimit=-2
      settings: AttributesFormatString="Min = %<LowerLimit>  Max = %<UpperLimit>"
  Saturation7 : Saturate  UpperLimit=2  LowerLimit=0.8
      settings: AttributesFormatString="Min = %<LowerLimit>  Max = %<UpperLimit>"
  Saturation8 : Saturate  UpperLimit=2  LowerLimit=0.8
      settings: AttributesFormatString="Min = %<LowerLimit>  Max = %<UpperLimit>"
  Saturation9 : Saturate  UpperLimit=2  LowerLimit=-2
      settings: AttributesFormatString="Min = %<LowerLimit>  Max = %<UpperLimit>"
  Unary Minus : UnaryMinus
  TTLCCalc_bsTTLCInfo : Outport
  tag scope: LFTTTLC_Mon=global, RGTTTLC_Mon=global
  wires:
  In4/1 -> Bus Selector3/1
  Bus Selector3/1 -> [CurL]  "<crPrvwCrvtLft>"
  Bus Selector3/2 -> [CurR]  "<crPrvwCrvtRgt>"
  Gain2/1 -> MATLAB Function5/1(vx), [Vx]
  Bus Selector4/7 -> Gain2/1  "<ESC_VehSpd>"
  bsLLClb/1 -> Bus Selector5/1
  bsInfo/1 -> Bus Selector4/1
  bsDvtInfo/1 -> Bus Selector2/1
  Bus Selector2/2 -> MATLAB Function1/1(dvt)  "<IRgtDvt>"
  [VxL0] -> MATLAB Function/2(vy)
  [VxR0] -> MATLAB Function1/2(vy)
  MATLAB Function1/1(TTLC) -> Saturation1/1  "RGTLC"
  MATLAB Function/1(TTLC) -> Saturation/1
  Saturation/1 -> [LftTTLC]  "LftTTLC"
  Saturation1/1 -> [RgtTTLC]  "RgtTTLC"
  Bus Selector2/1 -> MATLAB Function/1(dvt)  "<ILftDvt>"
  [CurR] -> MATLAB Function1/3(cur)
  [CurL] -> MATLAB Function/3(cur)
  Bus Selector4/5 -> [R0C1]  "<R0_C1>"
  Bus Selector4/4 -> [R0C0]  "<R0_C0>"
  Bus Selector4/6 -> [R0C2]  "<R0_C2>"
  Bus Selector4/2 -> [L0C1]  "<L0_C1>"
  Bus Selector4/1 -> [L0C0]  "<L0_C0>"
  Bus Selector4/3 -> [L0C2]  "<L0_C2>"
  [C20] -> MATLAB Function3/5(c20)
  MATLAB Function4/1(TRgt) -> [TRgt]  "TRgt"
  [R0C2] -> MATLAB Function4/3(c2)
  [Vx] -> MATLAB Function3/4(vx)
  [C20] -> MATLAB Function4/5(c20)
  [W] -> MATLAB Function4/6(w)
  [R0C0] -> MATLAB Function4/1(c0)
  MATLAB Function3/1(TLft) -> [TLft]  "TLft"
  [L0C1] -> MATLAB Function3/2(c1)
  [W] -> MATLAB Function3/6(w)
  [R0C1] -> MATLAB Function4/2(c1)
  [Vx] -> MATLAB Function4/4(vx)
  [L0C2] -> MATLAB Function3/3(c2)
  [L0C0] -> MATLAB Function3/1(c0)
  Product3/1 -> Saturation10/1  "V_R0"
  [Vx] -> Product3/1
  [L0C1] -> Product/2
  [Vx] -> Product/1
  Saturation9/1 -> [VxL0]  "VL0"
  Product/1 -> Unary Minus/1  "V_L0"
  [R0C1] -> Product3/2
  Unary Minus/1 -> Saturation9/1
  Saturation10/1 -> [VxR0]  "VR0"
  Bus Creator/1 -> TTLCCalc_bsTTLCInfo/1
  [TLft] -> MATLAB Function2/7(TLft)
  [LftTTLC] -> MATLAB Function2/5(LTTLC)
  [TRgt] -> MATLAB Function2/8(TRgt)
  Saturation7/1 -> [LFTTTLC_Mon], Bus Creator/1  "LFTTTLC"
  [CurL] -> MATLAB Function2/1(crPrvwCrvtLft)
  MATLAB Function2/1(LFTTTLC) -> Saturation7/1  "LFTTTLC"
  [RgtTTLC] -> MATLAB Function2/6(RTTLC)
  MATLAB Function2/2(RGTTTLC) -> Saturation8/1  "RGTTTLC"
  Saturation8/1 -> Bus Creator/2, [RGTTTLC_Mon]  "RGTTTLC"
  [CurR] -> MATLAB Function2/2(crPrvwCrvtRgt)
  Bus Selector4/8 -> Degrees to Radians/1  "<SW_Angle>"
  Degrees to Radians/1 -> MATLAB Function5/2(sw_angle)
  Bus Selector5/1 -> MATLAB Function5/3(WhlBaseL_C)  "<LKA_WhlBaseL_C>"
  MATLAB Function5/1(TTLC) -> [C20]
  Bus Selector5/3 -> [W]  "<LKA_Veh2CamW_C>"
  Bus Selector5/2 -> MATLAB Function5/4(StrRatio_C)  "<LKA_StrRatio_C>"
  [VxL0] -> Bus Creator/3  "vLft"
  [VxR0] -> Bus Creator/4  "vRgt"
  [LTLC] -> MATLAB Function2/3(LTLC)
  [RTLC] -> MATLAB Function2/4(RTLC)
  Constant/1 -> [LTLC]
  Constant1/1 -> [RTLC]

== system LKAS_AutoSave_20220223_1234/LKAS/LL/LLOn/LKA Input Processing (LKAInP)/Under The Limit (UndrLim) ==
  UndrLim_bsInInfoSyn : Inport
  UndrLim_bsLLClb : Inport  Port=2
  Bus Creator : BusCreator  Inputs=2
  Bus Selector1 : BusSelector  OutputSignals=bsVehMovInfo.ESC_VehSpd
  Bus Selector2 : BusSelector  OutputSignals=bsLKAClb.LL_LAccMax_C,bsLKAClb.LL_LAccRMax_C,bsConstantClb.LKA_StrRatio_C,bsConstantClb.LKA_WhlBaseL_C
  Saturation : Saturate  UpperLimit=150  LowerLimit=0.001
      settings: AttributesFormatString="Min = %<LowerLimit>  Max = %<UpperLimit>"
  Steering Wheel Angel Max (SWAMax) : Subsystem
  Steering Wheel Angel Rate Max (SWARMax) : Subsystem
  UndrLim_bsUndrLimInfo : Outport
  wires:
  Saturation/1 -> Steering Wheel Angel Rate Max (SWARMax)/1(SWARateMax_vVehSpd), Steering Wheel Angel Max (SWAMax)/1(SWAMax_vVehSpd)
  Steering Wheel Angel Rate Max (SWARMax)/1(SWARMax_dphiSWARMax) -> Bus Creator/2  "UndrLim_dphiSWARMax"
  Steering Wheel Angel Max (SWAMax)/1(SWAMax_phiSWAMax) -> Bus Creator/1  "UndrLim_phiSWAMax"
  UndrLim_bsInInfoSyn/1 -> Bus Selector1/1
  Bus Selector1/1 -> Saturation/1  "<ESC_VehSpd>"
  UndrLim_bsLLClb/1 -> Bus Selector2/1
  Bus Selector2/1 -> Steering Wheel Angel Max (SWAMax)/2(SWAMax_aLAcc_C)  "<LL_LAccMax_C>"
  Bus Selector2/2 -> Steering Wheel Angel Rate Max (SWARMax)/2(SWARateMax_aLAccR_C)  "<LL_LAccRMax_C>"
  Bus Selector2/3 -> Steering Wheel Angel Rate Max (SWARMax)/3(LKA_StrRatio_C), Steering Wheel Angel Max (SWAMax)/3(LKA_StrRatio_C)  "<LKA_StrRatio_C>"
  Bus Selector2/4 -> Steering Wheel Angel Max (SWAMax)/4(LKA_WhlBaseL_C), Steering Wheel Angel Rate Max (SWARMax)/4(LKA_WhlBaseL_C)  "<LKA_WhlBaseL_C>"
  Bus Creator/1 -> UndrLim_bsUndrLimInfo/1

== system LKAS_AutoSave_20220223_1234/LKAS/LL/LLOn/LL State Determination (LLStateDet)/LL State Machine Conditions (LLSMCon) ==
  LLSMCon_bsInInfoSyn : Inport
  LLSMCon_bsLKAInPInfo : Inport  Port=2
  LLSMCon_bsLLClb : Inport  Port=3
  LLSMCon_bsLLState : Inport  Port=4
  LLSMCon_stExitFlg : Inport  Port=5
  LLSMCon_bsSignalFault : Inport  Port=6
  Activation Condition (ActvC) : Subsystem  Description=|
      | Block Name: Activation Condition
      | Ab.: ActvC
      | No.: 1.1.1.4.0.
      | Rev: 0.0.1
      | Update Date: 19-3-26
  Bus Selector : BusSelector  OutputSignals=bsMP5Info.LKA_Mode
  Cast : DataTypeConversion
  Cast1 : DataTypeConversion
  Deactivation Condition (DeactvC) : Subsystem  Description=|
      | Block Name: Deactivation Condition
      | Ab.: DeactvC
      | No.: 1.1.1.5.0.0
      | Rev: 0.0.1
      | Update Date: 19-3-26
  Disable Condition (DisblC) : Subsystem  Description=|
      | Block Name: Disable Condition
      | Ab.: DisblC
      | No.: 1.1.1.3.0.0
      | Rev: 0.0.1
      | Update Date: 19-3-26
  Enable Condition (EnaC) : Subsystem  Description=|
      | Block Name: Enable Condition
      | Ab.: EnaC
      | No.: 1.1.1.2.0.0
      | Rev: 0.0.1
      | Update Date: 19-3-26
      settings: PermitHierarchicalResolution=None  MinAlgLoopOccurrences=on
  Fault Condition (FaultC) : Subsystem  Description=|
      | Block Name: Fault Condition
      | Ab.: FaultC
      | No.: 1.1.1.6.0.0
      | Rev: 0.0.1
      | Update Date: 19-3-26
  Terminator : Terminator
  Terminator1 : Terminator
  LLSMCon_stDACMode : Outport
  LLSMCon_stLDWEnaCSyn : Outport  Port=2
  LLSMCon_stLDWDisblCSyn : Outport  Port=3
  LLSMCon_stLDWActvCSyn : Outport  Port=4
  LLSMCon_stLDWDeactvCSyn : Outport  Port=5
  LLSMCon_stLDWFaultCSyn : Outport  Port=6
  LLSMCon_stLKAEnaCSyn : Outport  Port=7
  LLSMCon_stLKADisblCSyn : Outport  Port=8
  LLSMCon_stLKAActvCSyn : Outport  Port=9
  LLSMCon_stLKADeactvCSyn : Outport  Port=10
  LLSMCon_stLKAFaultCSyn : Outport  Port=11
  Disable_Reason : Outport  Port=12
  wires:
  Enable Condition (EnaC)/2(EnaC_stLKAEnaCSyn) -> LLSMCon_stLKAEnaCSyn/1
  Disable Condition (DisblC)/1(DisblC_stLDWDisblCSyn) -> LLSMCon_stLDWDisblCSyn/1
  Disable Condition (DisblC)/2(DisblC_stLKADisblCSyn) -> LLSMCon_stLKADisblCSyn/1
  Enable Condition (EnaC)/1(EnaC_stLDWEnaCSyn) -> LLSMCon_stLDWEnaCSyn/1
  LLSMCon_bsLLState/1 -> Deactivation Condition (DeactvC)/5(LLState), Disable Condition (DisblC)/5(LLState)
  LLSMCon_bsInInfoSyn/1 -> Bus Selector/1, Enable Condition (EnaC)/2(EnaC_bsInInfoSyn), Fault Condition (FaultC)/1(FaultC_bsInInfoSyn), Deactivation Condition (DeactvC)/2(InInfoSyn), Activation Condition (ActvC)/2(InInfoSyn), Disable Condition (DisblC)/2(InInfoSyn)
  Activation Condition (ActvC)/1(ActvC_stLDWActvCSyn) -> LLSMCon_stLDWActvCSyn/1
  Fault Condition (FaultC)/1(FaultC_stLDWFaultCSyn) -> LLSMCon_stLDWFaultCSyn/1
  Deactivation Condition (DeactvC)/2(DeactvC_stLKADeactvCSyn) -> LLSMCon_stLKADeactvCSyn/1, Cast1/1
  Fault Condition (FaultC)/2(FaultC_stLKAFaultCSyn) -> LLSMCon_stLKAFaultCSyn/1
  Deactivation Condition (DeactvC)/1(DeactvC_stLDWDeactvCSyn) -> LLSMCon_stLDWDeactvCSyn/1
  LLSMCon_stExitFlg/1 -> Deactivation Condition (DeactvC)/6(ExitFlg)
  LLSMCon_bsLLClb/1 -> Fault Condition (FaultC)/2(FaultC_bsLLClb), Deactivation Condition (DeactvC)/4(LLClb), Activation Condition (ActvC)/4(LLClb), Disable Condition (DisblC)/4(LLClb), Enable Condition (EnaC)/4(EnaC_bsLLClb)
  Activation Condition (ActvC)/2(ActvC_stLKAActvCSyn) -> LLSMCon_stLKAActvCSyn/1
  LLSMCon_bsSignalFault/1 -> Fault Condition (FaultC)/3(FaultC_SignalFault)
  LLSMCon_bsLKAInPInfo/1 -> Deactivation Condition (DeactvC)/3(LKAInPInfo), Activation Condition (ActvC)/3(LKAInPInfo), Disable Condition (DisblC)/3(LKAInPInfo), Enable Condition (EnaC)/3(EnaC_bsLKAInPInfo)
  Bus Selector/1 -> Deactivation Condition (DeactvC)/1(DACMode), Activation Condition (ActvC)/1(DACMode), Disable Condition (DisblC)/1(DACMode), Enable Condition (EnaC)/1(EnaC_stDACMode), LLSMCon_stDACMode/1  "<LKA_Mode>"
  Cast/1 -> Terminator/1  "ob_LKA_Disable_Reason"
  Disable Condition (DisblC)/3(Disable_Reason) -> Disable_Reason/1, Cast/1  "Disable_Reason"
  Cast1/1 -> Terminator1/1  "ob_LKA_LKADeactvCSyn"

== system LKAS_AutoSave_20220223_1234/LKAS/LL/LLOut/Angle2Trq/Rate Limiter Dynamic ==
  note: U(k)
  note: Y(k)
  up : Inport
  u : Inport  Port=2
  lo : Inport  Port=3
  Delay Input2 : UnitDelay  Description=Store in Global RAM  DisableCoverage=on  SampleTime=-1
  Difference Inputs1 : Sum  Description=Add in CPU  DisableCoverage=on  Inputs=+-  OutDataTypeStr=Inherit: Inherit via back propagation
  Difference Inputs2 : Sum  Description=Add in CPU  OutDataTypeStr=Inherit: Inherit via back propagation
  FixPt Data Type Duplicate : DataTypeDuplicate  DisableCoverage=on  NumInputPorts=7
  Saturation Dynamic : simulink/Discontinuities/Saturation Dynamic  OutMin=[]  OutMax=[]  OutDataTypeStr=Inherit: Same as second input  OutDataType=fixdt(1, 16)  OutScaling=2^-10  DoSatur=off
  delta fall limit : Product  DisableCoverage=on  Inputs=**  OutDataTypeStr=Inherit: Inherit via back propagation  SaturateOnIntegerOverflow=on
  delta rise limit : Product  DisableCoverage=on  Inputs=**  OutDataTypeStr=Inherit: Inherit via back propagation  SaturateOnIntegerOverflow=on
  sample time : SampleTimeMath  DisableCoverage=on  TsampMathOp=Ts Only  weightValue=1
  Y : Outport  InitialOutput=0
  wires:
  u/1 -> sample time/1, FixPt Data Type Duplicate/5, Difference Inputs1/1
  delta fall limit/1 -> Saturation Dynamic/3, FixPt Data Type Duplicate/3
  up/1 -> delta rise limit/1
  sample time/1 -> delta rise limit/2, delta fall limit/2
  Saturation Dynamic/1 -> FixPt Data Type Duplicate/7, Difference Inputs2/1
  delta rise limit/1 -> Saturation Dynamic/1, FixPt Data Type Duplicate/6
  Difference Inputs1/1 -> Saturation Dynamic/2, FixPt Data Type Duplicate/4  "( U(k) - Y(k-1) )"
  lo/1 -> delta fall limit/1
  Delay Input2/1 -> Difference Inputs2/2, FixPt Data Type Duplicate/2, Difference Inputs1/2  "Y(k-1)"
  Difference Inputs2/1 -> FixPt Data Type Duplicate/1, Delay Input2/1, Y/1

== system LKAS_AutoSave_20220223_1234/LKAS/LL/LLOut/Angle2Trq/Saturation Dynamic ==
  up : Inport
  u : Inport  Port=2
  lo : Inport  Port=3
  Data Type Duplicate : DataTypeDuplicate  DisableCoverage=on
  Data Type Propagation : simulink/Signal Attributes/Data Type Propagation  PropDataType=fixdt(1, 16)  IfRefDouble=double  IfRefSingle=single  IsSigned=IsSigned1  NumBitsBase=NumBits1  NumBitsMult=1  NumBitsAdd=0  NumBitsAllowFinal=1:128  PropScaling=2^-10  ValuesUsedBestPrec=[5 -7]  SlopeBase=Slope1  SlopeMult=1  SlopeAdd=0  BiasBase=Bias1  BiasMult=1  BiasAdd=0
      settings: SourceProductName=Simulink  SourceProductBaseCode=SL
  LowerRelop1 : RelationalOperator  DisableCoverage=on  Operator=>  OutDataTypeStr=boolean  RndMeth=Nearest
  Switch : Switch  Criteria=u2 ~= 0  OutDataTypeStr=Inherit: Inherit via back propagation  ZeroCross=off
  Switch2 : Switch  Criteria=u2 ~= 0  OutDataTypeStr=Inherit: Inherit via back propagation  ZeroCross=off
  UpperRelop : RelationalOperator  DisableCoverage=on  Operator=<  OutDataTypeStr=boolean  RndMeth=Nearest
  y : Outport
  wires:
  LowerRelop1/1 -> Switch2/2
  Switch2/1 -> Data Type Duplicate/1, y/1
  lo/1 -> UpperRelop/2, Switch/1
  up/1 -> LowerRelop1/2, Switch2/1
  u/1 -> UpperRelop/1, Switch/3, LowerRelop1/1, Data Type Propagation/1, Data Type Propagation/2
  UpperRelop/1 -> Switch/2
  Switch/1 -> Data Type Propagation/3, Switch2/3, Data Type Duplicate/2

== system LKAS_AutoSave_20220223_1234/LKAS/LL/LLOut/Angle2Trq/Subsystem ==
  Target_Angle : Inport
  Stearing_Angle : Inport  Port=2
  Enable : EnablePort  StatesWhenEnabling=reset
  Add : Sum  Inputs=+-
  Add1 : Sum
  Add2 : Sum  Inputs=+++
  Delay1 : Delay  DelayLength=1
  Fcn : Fcn  Expr=u(1)*u(1)*u(1)*0.000002+u(1)*u(1)*(-0.0005)+u(1)*0.0505
  Ki : Constant  Value=0.0005  OutDataTypeStr=single
  Kp : Constant  Value=0.02  OutDataTypeStr=single
  Product1 : Product
  Product2 : Product
  Saturation : Saturate
  in_trq : Outport  OutputWhenDisabled=reset  InitialOutput=0
  wires:
  Add1/1 -> Saturation/1
  Target_Angle/1 -> Add/1, Fcn/1
  Product1/1 -> Add2/2  "Kp"
  Kp/1 -> Product1/2
  Delay1/1 -> Add1/2
  Saturation/1 -> Delay1/1, Add2/3  "Ki"
  Product2/1 -> Add1/1
  Add/1 -> Product2/1, Product1/1  "derta_angle"
  Ki/1 -> Product2/2
  Fcn/1 -> Add2/1  "Kf"
  Add2/1 -> in_trq/1  "in_trq"
  Stearing_Angle/1 -> Add/2

== system LKAS_AutoSave_20220223_1234/LKAS/LL/LL Inputs Mapping/bsLaneInfo/LaneSelect/Subsystem ==
  R0_Q_In : Inport
  Constant1 : Constant  Value=3  OutDataTypeStr=uint8
  Switch1 : Switch  Threshold=2
  R0_Q : Outport
  wires:
  Switch1/1 -> R0_Q/1  "R0_Q"
  R0_Q_In/1 -> Switch1/3, Switch1/2
  Constant1/1 -> Switch1/1

== system LKAS_AutoSave_20220223_1234/LKAS/LL/LL Inputs Mapping/bsLaneInfo/LaneSelect/Subsystem1 ==
  L1_Q_In : Inport
  Constant1 : Constant  Value=3  OutDataTypeStr=uint8
  Switch1 : Switch  Threshold=2
  L1_Q : Outport
  wires:
  Constant1/1 -> Switch1/1
  L1_Q_In/1 -> Switch1/2, Switch1/3
  Switch1/1 -> L1_Q/1  "L1_Q"

== system LKAS_AutoSave_20220223_1234/LKAS/LL/LL Inputs Mapping/bsLaneInfo/LaneSelect/Subsystem2 ==
  R1_Q_In : Inport
  Constant1 : Constant  Value=3  OutDataTypeStr=uint8
  Switch1 : Switch  Threshold=2
  R1_Q : Outport
  wires:
  Switch1/1 -> R1_Q/1  "R1_Q"
  R1_Q_In/1 -> Switch1/3, Switch1/2
  Constant1/1 -> Switch1/1

== system LKAS_AutoSave_20220223_1234/LKAS/LL/LL Inputs Mapping/bsLaneInfo/LaneSelect/Subsystem4 ==
  L0_Q_In : Inport
  Constant : Constant  Value=3  OutDataTypeStr=uint8
  Switch : Switch  Threshold=2
  L0_Q : Outport
  wires:
  Switch/1 -> L0_Q/1  "L0_Q"
  Constant/1 -> Switch/1
  L0_Q_In/1 -> Switch/2, Switch/3

== system LKAS_AutoSave_20220223_1234/LKAS/LL/LL Inputs Mapping/bsLaneInfo/LanesReconstruct /Left 1Lane Reconstruct (Lft1LaneR) ==
  stFlag : Inport
  bsL1Info : Inport  Port=2
  Bus Creator2 : BusCreator  Inputs=8
  Bus Selector1 : BusSelector  OutputSignals=L1_C0,L1_C1,L1_C2,L1_C3,L1_VR,L1_Q,L1_Type,L1_W
  Constant : Constant  Value=0  OutDataTypeStr=uint16
  Switch3 : Switch  Criteria=u2 > Threshold
  bsL1InfoR : Outport
  wires:
  Bus Selector1/8 -> Bus Creator2/8  "<L1_W>"
  Bus Selector1/7 -> Bus Creator2/7  "<L1_Type>"
  Bus Selector1/5 -> Bus Creator2/5  "<L1_VR>"
  bsL1Info/1 -> Bus Selector1/1
  stFlag/1 -> Switch3/2
  Bus Selector1/6 -> Switch3/1  "<L1_Q>"
  Constant/1 -> Switch3/3
  Switch3/1 -> Bus Creator2/6  "L1_Q"
  Bus Creator2/1 -> bsL1InfoR/1  "bsL1Info"
  Bus Selector1/4 -> Bus Creator2/4  "<L1_C3>"
  Bus Selector1/3 -> Bus Creator2/3  "<L1_C2>"
  Bus Selector1/2 -> Bus Creator2/2  "<L1_C1>"
  Bus Selector1/1 -> Bus Creator2/1  "<L1_C0>"

== system LKAS_AutoSave_20220223_1234/LKAS/LL/LL Inputs Mapping/bsLaneInfo/LanesReconstruct /Left Lane Reconstruct (LftLaneR) ==
  lRoadW : Inport
  bsR0Info : Inport  Port=2
  bsL0Info : Inport  Port=3
  Add : Sum  Inputs=+-  OutDataTypeStr=single
  Bus Creator : BusCreator  Inputs=8
  Bus Selector1 : BusSelector  OutputSignals=L0_Q
  Bus Selector3 : BusSelector  OutputSignals=R0_C0,R0_C1,R0_C2,R0_C3,R0_VR,R0_Type,R0_W
  Cast To Single{1..4,6} (5 alike) : DataTypeConversion  OutDataTypeStr=single  LockScale=on
  Cast To Single5 : DataTypeConversion  OutDataTypeStr=uint8  LockScale=on
  Gain : Gain  Gain=-1  OutDataTypeStr=Inherit: Same as input
  bsL0InfoR : Outport
  wires:
  Cast To Single4/1 -> Bus Creator/5  "L0_VR"
  Cast To Single6/1 -> Bus Creator/8  "L0_W"
  Cast To Single5/1 -> Bus Creator/7  "L0_Type"
  Bus Selector3/7 -> Cast To Single6/1  "<R0_W>"
  Bus Selector3/6 -> Cast To Single5/1  "<R0_Type>"
  lRoadW/1 -> Add/1
  bsR0Info/1 -> Bus Selector3/1
  Bus Selector3/1 -> Add/2  "<R0_C0>"
  Add/1 -> Gain/1
  Bus Selector3/2 -> Cast To Single1/1  "<R0_C1>"
  Bus Selector3/3 -> Cast To Single2/1  "<R0_C2>"
  Bus Selector3/4 -> Cast To Single3/1  "<R0_C3>"
  Bus Selector3/5 -> Cast To Single4/1  "<R0_VR>"
  bsL0Info/1 -> Bus Selector1/1
  Bus Selector1/1 -> Bus Creator/6  "<L0_Q>"
  Gain/1 -> Bus Creator/1  "L0_C0"
  Cast To Single1/1 -> Bus Creator/2  "L0_C1"
  Cast To Single2/1 -> Bus Creator/3  "L0_C2"
  Cast To Single3/1 -> Bus Creator/4  "L0_C3"
  Bus Creator/1 -> bsL0InfoR/1  "bsL0Info"

== system LKAS_AutoSave_20220223_1234/LKAS/LL/LL Inputs Mapping/bsLaneInfo/LanesReconstruct /Right 1Lane Reconstruct (Rgt1LaneR) ==
  stFlag : Inport
  bsR1Info : Inport  Port=2
  Bus Creator3 : BusCreator  Inputs=8
  Bus Selector1 : BusSelector  OutputSignals=R1_C0,R1_C1,R1_C2,R1_C3,R1_VR,R1_Q,R1_Type,R1_W
  Constant : Constant  Value=0  OutDataTypeStr=uint16
  Switch3 : Switch  Criteria=u2 > Threshold
  bsL1InfoR : Outport
  wires:
  Bus Selector1/8 -> Bus Creator3/8  "<R1_W>"
  Bus Selector1/7 -> Bus Creator3/7  "<R1_Type>"
  Bus Selector1/5 -> Bus Creator3/5  "<R1_VR>"
  Bus Selector1/1 -> Bus Creator3/1  "<R1_C0>"
  Bus Selector1/2 -> Bus Creator3/2  "<R1_C1>"
  Bus Selector1/3 -> Bus Creator3/3  "<R1_C2>"
  Bus Selector1/4 -> Bus Creator3/4  "<R1_C3>"
  Constant/1 -> Switch3/3
  Bus Selector1/6 -> Switch3/1  "<R1_Q>"
  stFlag/1 -> Switch3/2
  bsR1Info/1 -> Bus Selector1/1
  Bus Creator3/1 -> bsL1InfoR/1  "bsR1Info"
  Switch3/1 -> Bus Creator3/6  "R1_Q"
